simulink model "Battery_model_in_Simulink"  (R2022b)
settings: Solver=VariableStepAuto  StartTime=0.0  StopTime=6.5  RelTol=1e-3
undefined symbols (not defined in the file or in its folder): bp
settings Model: Creator=harry  LastModifiedBy=harry

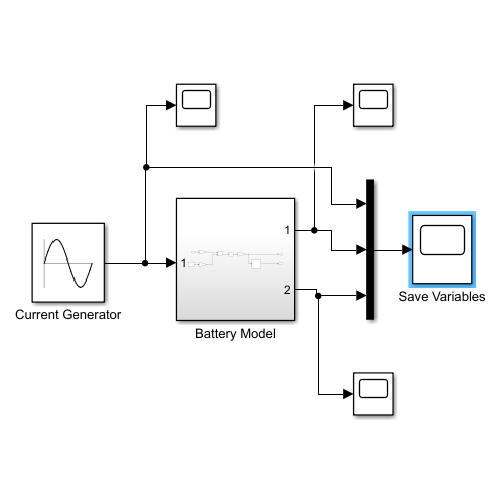
[thumbnail: Simulink's stored preview of the top-level diagram]
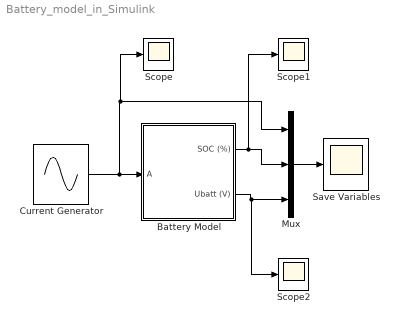
== system Battery_model_in_Simulink ==
  Battery Model : Subsystem
  Current Generator : Sin  Amplitude=100  SampleTime=0
  Mux : Mux  Inputs=3
  Save Variables : Scope
  Scope : Scope
  Scope1 : Scope
  Scope2 : Scope
  wires:
  Current Generator/1 -> Scope/1, Mux/1, Battery Model/1(A)
  Battery Model/1(SOC (%)) -> Scope1/1, Mux/2
  Battery Model/2(Ubatt (V)) -> Scope2/1, Mux/3
  Mux/1 -> Save Variables/1

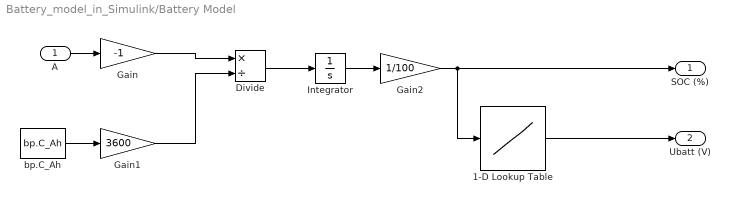
== system Battery_model_in_Simulink/Battery Model ==
  A : Inport
  1-D Lookup Table : Lookup_n-D  NumberOfTableDimensions=1  BreakpointsForDimension1=bp.SOC_x_pct  Table=bp.U_y_V  InternalRulePriority=Speed  RndMeth=Simplest
  Divide : Product  Inputs=*/
  Gain : Gain  Gain=-1
  Gain1 : Gain  Gain=3600
  Gain2 : Gain  Gain=1/100
  Integrator : Integrator  InitialCondition=bp.SOC0_pct
  bp.C_Ah : Constant  Value=bp.C_Ah
  SOC (%) : Outport
  Ubatt (V) : Outport  Port=2
  wires:
  Integrator/1 -> Gain2/1
  Gain1/1 -> Divide/2
  bp.C_Ah/1 -> Gain1/1
  Divide/1 -> Integrator/1
  Gain2/1 -> SOC (%)/1, 1-D Lookup Table/1
  Gain/1 -> Divide/1
  1-D Lookup Table/1 -> Ubatt (V)/1
  A/1 -> Gain/1
